simulink model "model_8264"  (R2022b)
settings: Solver=FixedStepAuto  StartTime=0.0  StopTime=2.4  FixedStep=2e-5  RelTol=1e-3
undefined symbols (not defined in the file): Acid, Lead, sigbuilder_block
libraries: spsMeanLib x24, spsVoltageMeasurementLib x18, spsGroundLib x15, spsCurrentMeasurementLib x15, spsIdealSwitchLib x12, spsSeriesRLCLoadLib x12, spsSeriesRLCBranchLib x5, spsThreePhaseVIMeasurementLib x4, simulink x4, spsPower3phInstantaneousLib x3, spsThreePhaseBreakerLib x2, slpidlib x2
(part 1 of 2)
settings Model: Creator=LiChao  LastModifiedBy=ldt20
settings ModelReferenceCC: EnableRefExpFcnMdlSchedulingChecks=on

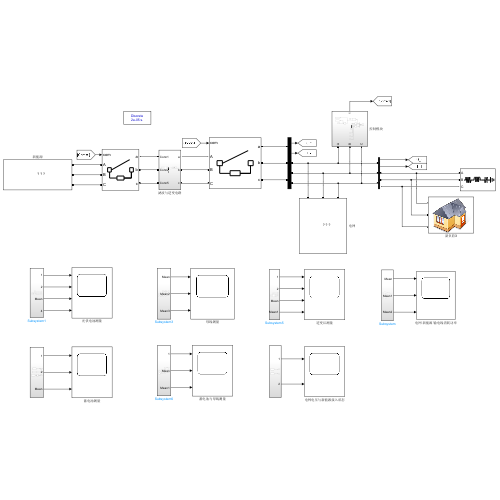
[thumbnail: Simulink's stored preview of the top-level diagram]
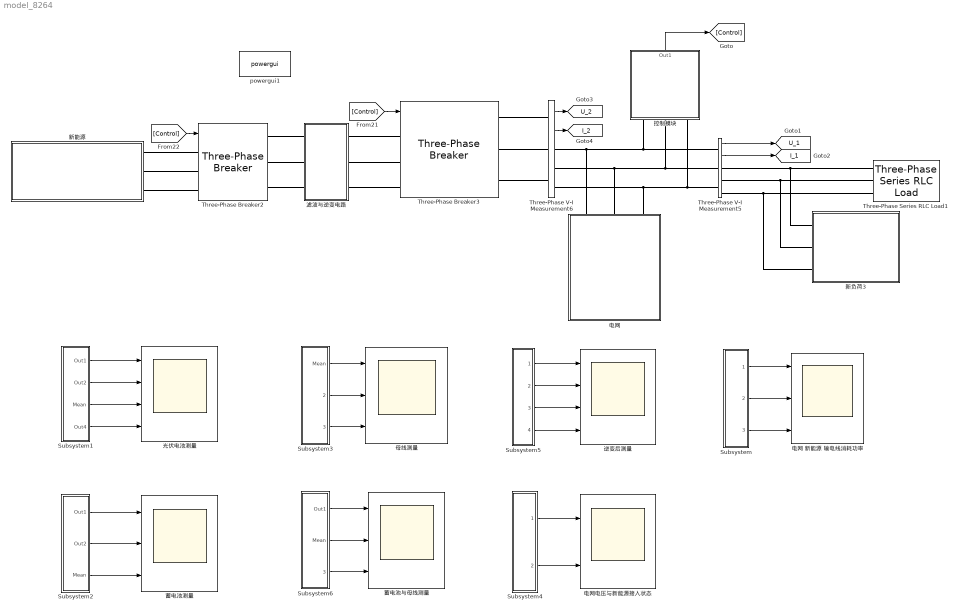
== system model_8264 ==
  Subsystem : Subsystem
  Subsystem1 : Subsystem
  Subsystem2 : Subsystem
  Subsystem3 : Subsystem
  Subsystem4 : Subsystem
  Subsystem5 : Subsystem
  Subsystem6 : Subsystem
  Three-Phase Series RLC Load1 : spsThreePhaseSeriesRLCLoadLib/Three-Phase Series RLC Load  LConnTagsString=A|B|C  Configuration=Y (grounded)  NominalVoltage=1000  Vabc=[1e3 1e3 1e3]  Vabcp=[1e3 1e3 1e3]  NominalFrequency=50  UnbalancedPower=off  ActivePower=1  InductivePower=100  CapacitivePower=100  Pabc=[10e3 9e3 11e3]  QLabc=[100 90 110]  QCabc=[100 90 110]  Pabcp=[10e3 9e3 11e3]  QLabcp=[100 90 110]  QCabcp=[100 90 110]  Measurements=None  LoadType=constant Z
  Three-Phase V-I Measurement5 : spsThreePhaseVIMeasurementLib/Three-Phase V-I Measurement  VoltageMeasurement=phase-to-ground  SetLabelV=off  LabelV=Vgrid0  Vpu=off  VpuLL=off  CurrentMeasurement=yes  SetLabelI=off  LabelI=Igrid  Ipu=off  Pbase=100e6  Vbase=500e3  OutputType=Complex  PhasorSimulation=off  PSBequivalent=0
  Three-Phase V-I Measurement6 : spsThreePhaseVIMeasurementLib/Three-Phase V-I Measurement  VoltageMeasurement=phase-to-ground  SetLabelV=off  LabelV=Vgrid0  Vpu=off  VpuLL=off  CurrentMeasurement=yes  SetLabelI=off  LabelI=Igrid  Ipu=off  Pbase=100e6  Vbase=500e3  OutputType=Complex  PhasorSimulation=off  PSBequivalent=0
  Three-Phase Breaker2 : spsThreePhaseBreakerLib/Three-Phase Breaker  InitialState=open  SwitchA=on  SwitchB=on  SwitchC=on  SwitchTimes="[1/60  5/60]"  External=on  BreakerResistance=0.01  SnubberResistance=1e6  SnubberCapacitance=inf  Measurements=None
  Three-Phase Breaker3 : spsThreePhaseBreakerLib/Three-Phase Breaker  InitialState=open  SwitchA=on  SwitchB=on  SwitchC=on  SwitchTimes="[1/60  5/60]"  External=on  BreakerResistance=0.01  SnubberResistance=1e6  SnubberCapacitance=inf  Measurements=None
  powergui1 : spspowerguiLib/powergui  Priority=1  SimulationMode=Discrete  SampleTime=2e-5  frequency=60  Iterations=50  frequencyindice=0  Pbase=100e6  ErrMax=1e-4  UnitsV=kV  UnitsW=MW  buscounter=0  FunctionMessages=off  echomessages=off  EnableUseOfTLC=off  CurrentSourceSwitches=off  DisableSnubberDevices=off  DisableRonSwitches=off  DisableVfSwitches=off  DisplayEquations=off  AutomaticDiscreteSolvers=off  SolverType=Tustin/Backward Euler (TBE)  Interpol=off  ExternalGateDelay=off  methode=off  Ts=100  x0status=blocks  SPID=on  SwTol=0  HookPort=off  NonlinearTolerance=1e-4  nMaxIteration=100  ContinueOnMaxIteration=off  RestoreLinks=warning  ResistiveCurrentMeasurement=off  Frange=[0:2:500]  Ylog=off  Xlog=on  ShowGrid=off  save=off  variable=ZData  structure=0  ZoomFFT=off  StartTime=0.0  cycles=1  DisplayStyle=1  fundamental=60  FreqAxis=off  MaxFrequency=1000  frequencyindicesteady=1  RmsSteady=1  display=off
  光伏电池测量 : Scope  NumInputPorts=4
  控制模块 : Subsystem
  新能源 : Subsystem
      mask Display: image('xinengyuan.jpg'); % 使用工具条上的 "编辑图像" 进行更改。
  新负荷3 : Subsystem
      mask Display: image('house.jpg'); % 使用工具条上的 "编辑图像" 进行更改。
  母线测量 : Scope  NumInputPorts=3
  滤波与逆变电路 : Subsystem
  电网 : Subsystem
      mask Display: image('dianwang.jpg'); % 使用工具条上的 "编辑图像" 进行更改。
  电网 新能源 输电线消耗功率 : Scope  NumInputPorts=3
  电网电压与新能源接入状态 : Scope  NumInputPorts=2
  蓄电池与母线测量 : Scope  NumInputPorts=3
  蓄电池测量 : Scope  NumInputPorts=3
  逆变后测量 : Scope  NumInputPorts=4
  tag scope: I_1=global, I_2=global, U_1=global, U_2=global
  wires:
  控制模块/1(Out1) -> [Control]
  [Control] -> Three-Phase Breaker3/1
  [Control] -> Three-Phase Breaker2/1
  Three-Phase V-I Measurement5/1 -> [U_1]
  Three-Phase V-I Measurement5/2 -> [I_1]
  Three-Phase V-I Measurement6/1 -> [U_2]
  Three-Phase V-I Measurement6/2 -> [I_2]
  Subsystem/1(Mean) -> 电网 新能源 输电线消耗功率/1
  Subsystem/2(Mean1) -> 电网 新能源 输电线消耗功率/2
  Subsystem/3(Mean2) -> 电网 新能源 输电线消耗功率/3
  Subsystem1/1(Out1) -> 光伏电池测量/1
  Subsystem1/2(Out2) -> 光伏电池测量/2
  Subsystem1/3(Mean) -> 光伏电池测量/3
  Subsystem1/4(Out4) -> 光伏电池测量/4
  Subsystem2/1(Out1) -> 蓄电池测量/1
  Subsystem2/2(Out2) -> 蓄电池测量/2
  Subsystem2/3(Mean) -> 蓄电池测量/3
  Subsystem3/1(Mean) -> 母线测量/1
  Subsystem3/2(Mean2) -> 母线测量/2
  Subsystem3/3(Mean3) -> 母线测量/3
  Subsystem4/1(Out1) -> 电网电压与新能源接入状态/1
  Subsystem4/2(Out2) -> 电网电压与新能源接入状态/2
  Subsystem5/1(Out1) -> 逆变后测量/1
  Subsystem5/2(Out2) -> 逆变后测量/2
  Subsystem5/3(Mean) -> 逆变后测量/3
  Subsystem5/4(Mean1) -> 逆变后测量/4
  Subsystem6/1(Out1) -> 蓄电池与母线测量/1
  Subsystem6/2(Mean) -> 蓄电池与母线测量/2
  Subsystem6/3(Mean1) -> 蓄电池与母线测量/3
  connections:
  Three-Phase Breaker3/LConn1 -- 滤波与逆变电路/RConn1
  Three-Phase Breaker2/RConn2 -- 滤波与逆变电路/LConn2
  Three-Phase Breaker3/LConn2 -- 滤波与逆变电路/RConn2
  新能源/LConn1 -- Three-Phase Breaker2/LConn1
  Three-Phase Breaker3/LConn3 -- 滤波与逆变电路/RConn3
  新能源/LConn2 -- Three-Phase Breaker2/LConn2
  Three-Phase Breaker2/RConn3 -- 滤波与逆变电路/LConn3
  Three-Phase V-I Measurement6/LConn2 -- Three-Phase Breaker3/RConn2
  新能源/LConn3 -- Three-Phase Breaker2/LConn3
  Three-Phase V-I Measurement6/LConn3 -- Three-Phase Breaker3/RConn3
  Three-Phase Breaker2/RConn1 -- 滤波与逆变电路/LConn1
  Three-Phase V-I Measurement6/LConn1 -- Three-Phase Breaker3/RConn1
  Three-Phase V-I Measurement6/RConn1 -- 电网/RConn1 -- 控制模块/LConn1 -- Three-Phase V-I Measurement5/LConn1
  Three-Phase V-I Measurement6/RConn2 -- 电网/RConn2 -- 控制模块/LConn2 -- Three-Phase V-I Measurement5/LConn2
  Three-Phase V-I Measurement6/RConn3 -- 电网/RConn3 -- Three-Phase V-I Measurement5/LConn3 -- 控制模块/LConn3
  Three-Phase V-I Measurement5/RConn1 -- 新负荷3/LConn1 -- Three-Phase Series RLC Load1/LConn1
  Three-Phase V-I Measurement5/RConn2 -- 新负荷3/LConn2 -- Three-Phase Series RLC Load1/LConn2
  Three-Phase V-I Measurement5/RConn3 -- 新负荷3/LConn3 -- Three-Phase Series RLC Load1/LConn3

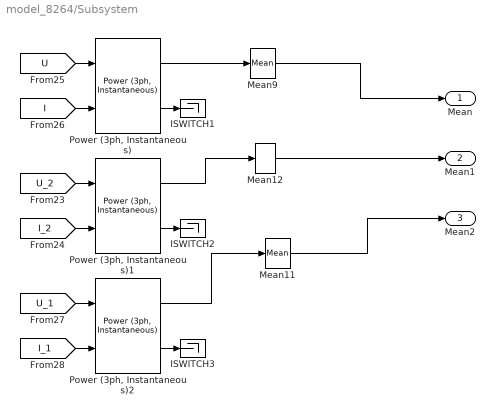
== system model_8264/Subsystem ==
  ISWITCH1 : Terminator
  ISWITCH2 : Terminator
  ISWITCH3 : Terminator
  Mean11 : spsMeanLib/Mean  Freq=50  Vinit=0  Ts=0
  Mean12 : spsMeanLib/Mean  Freq=50  Vinit=0  Ts=0
  Mean9 : spsMeanLib/Mean  Freq=50  Vinit=0  Ts=0
  "Power (3ph, Instantaneous)" : spsPower3phInstantaneousLib/Power (3ph, Instantaneous)
  "Power (3ph, Instantaneous)1" : spsPower3phInstantaneousLib/Power (3ph, Instantaneous)
  "Power (3ph, Instantaneous)2" : spsPower3phInstantaneousLib/Power (3ph, Instantaneous)
  Mean : Outport
  Mean1 : Outport  Port=2
  Mean2 : Outport  Port=3
  wires:
  Mean11/1 -> Mean2/1
  [I_1] -> "Power (3ph, Instantaneous)2"/2
  "Power (3ph, Instantaneous)2"/1 -> Mean11/1
  [U_2] -> "Power (3ph, Instantaneous)1"/1
  "Power (3ph, Instantaneous)1"/1 -> Mean12/1
  [U_1] -> "Power (3ph, Instantaneous)2"/1
  Mean12/1 -> Mean1/1
  [U] -> "Power (3ph, Instantaneous)"/1
  "Power (3ph, Instantaneous)"/1 -> Mean9/1
  [I] -> "Power (3ph, Instantaneous)"/2
  [I_2] -> "Power (3ph, Instantaneous)1"/2
  "Power (3ph, Instantaneous)2"/2 -> ISWITCH3/1
  "Power (3ph, Instantaneous)1"/2 -> ISWITCH2/1
  Mean9/1 -> Mean/1
  "Power (3ph, Instantaneous)"/2 -> ISWITCH1/1

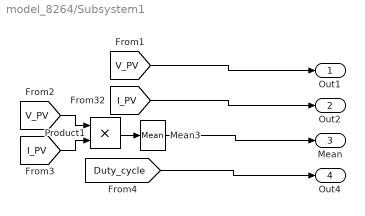
== system model_8264/Subsystem1 ==
  Mean3 : spsMeanLib/Mean  Freq=50  Vinit=0  Ts=0
  Product1 : Product
  Out1 : Outport
  Out2 : Outport  Port=2
  Mean : Outport  Port=3
  Out4 : Outport  Port=4
  wires:
  Product1/1 -> Mean3/1
  [V_PV] -> Product1/1
  Mean3/1 -> Mean/1
  [I_PV] -> Out2/1
  [Duty_cycle] -> Out4/1
  [I_PV] -> Product1/2
  [V_PV] -> Out1/1

== system model_8264/Subsystem2 ==
  Mean7 : spsMeanLib/Mean  Freq=50  Vinit=0  Ts=0
  Out1 : Outport
  Out2 : Outport  Port=2
  Mean : Outport  Port=3
  wires:
  [I_battery] -> Mean7/1
  [SOC] -> Out1/1
  Mean7/1 -> Mean/1
  [U_battery] -> Out2/1

== system model_8264/Subsystem3 ==
  Mean1 : spsMeanLib/Mean  Freq=50  Vinit=0  Ts=0
  Mean6 : spsMeanLib/Mean  Freq=50  Vinit=0  Ts=0
  Mean8 : spsMeanLib/Mean  Freq=50  Vinit=0  Ts=0
  Product2 : Product
  Mean : Outport
  Mean2 : Outport  Port=2
  Mean3 : Outport  Port=3
  wires:
  [I_BUS] -> Mean8/1
  [U_BUS] -> Mean6/1
  Mean8/1 -> Mean2/1
  [I_BUS] -> Product2/2
  Mean6/1 -> Mean/1
  Product2/1 -> Mean1/1
  [U_BUS] -> Product2/1
  Mean1/1 -> Mean3/1

== system model_8264/Subsystem4 ==
  Out1 : Outport
  Out2 : Outport  Port=2
  wires:
  [Grid_voltage] -> Out1/1
  [State] -> Out2/1

== system model_8264/Subsystem5 ==
  Mean4 : spsMeanLib/Mean  Freq=50  Vinit=0  Ts=0
  Mean5 : spsMeanLib/Mean  Freq=50  Vinit=0  Ts=0
  "Power (3ph, Phasor)2" : spsPower3phPhasorLib/Power (3ph, Phasor)
  Out1 : Outport
  Out2 : Outport  Port=2
  Mean : Outport  Port=3
  Mean1 : Outport  Port=4
  wires:
  Mean5/1 -> Mean1/1
  [U_ABC] -> "Power (3ph, Phasor)2"/1
  [I_ABC] -> Out2/1
  [I_ABC] -> "Power (3ph, Phasor)2"/2
  "Power (3ph, Phasor)2"/1 -> Mean4/1
  "Power (3ph, Phasor)2"/2 -> Mean5/1
  [U_ABC] -> Out1/1
  Mean4/1 -> Mean/1

== system model_8264/Subsystem6 ==
  Mean10 : spsMeanLib/Mean  Freq=50  Vinit=0  Ts=0
  Mean2 : spsMeanLib/Mean  Freq=50  Vinit=0  Ts=0
  Product3 : Product
  Out1 : Outport
  Mean : Outport  Port=2
  Mean1 : Outport  Port=3
  wires:
  [I_CM] -> Product3/2
  [U_BUS] -> Product3/1
  Product3/1 -> Mean2/1
  [I_CM] -> Mean10/1
  Mean2/1 -> Mean1/1
  Mean10/1 -> Mean/1
  [U_BUS] -> Out1/1

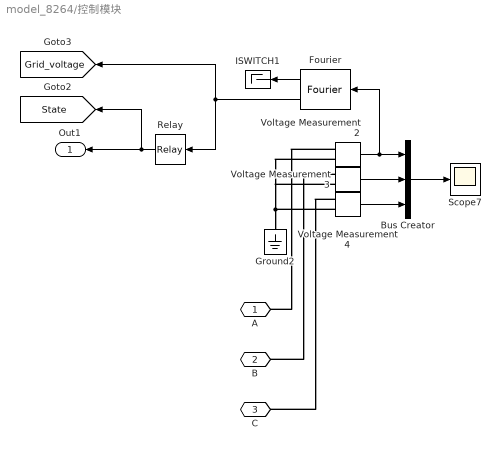
== system model_8264/控制模块 ==
  Bus Creator : BusCreator  Inputs=3
  Fourier : spsFourierLib/Fourier  Freq=50  n=1  InInit=[0, 0]  Ts=0
  Ground2 : spsGroundLib/Ground  LConnTagsString=a
  ISWITCH1 : Terminator
  Relay : Relay  OnSwitchValue=218  OffSwitchValue=215  OnOutputValue=0  OffOutputValue=1
  Scope7 : Scope
  Voltage Measurement2 : spsVoltageMeasurementLib/Voltage Measurement  PhasorSimulation=off  OutputType=Complex  PSBequivalent=0
  Voltage Measurement3 : spsVoltageMeasurementLib/Voltage Measurement  PhasorSimulation=off  OutputType=Complex  PSBequivalent=0
  Voltage Measurement4 : spsVoltageMeasurementLib/Voltage Measurement  PhasorSimulation=off  OutputType=Complex  PSBequivalent=0
  A : PMIOPort  Side=Left
  B : PMIOPort  Port=2  Side=Left
  C : PMIOPort  Port=3  Side=Left
  Out1 : Outport
  tag scope: Grid_voltage=global, State=global
  wires:
  Voltage Measurement2/1 -> Fourier/1, Bus Creator/1
  Fourier/2 -> ISWITCH1/1
  Bus Creator/1 -> Scope7/1
  Relay/1 -> [State], Out1/1
  Fourier/1 -> [Grid_voltage], Relay/1
  Voltage Measurement4/1 -> Bus Creator/3
  Voltage Measurement3/1 -> Bus Creator/2
  connections:
  Voltage Measurement4/LConn2 -- Voltage Measurement2/LConn2 -- Voltage Measurement3/LConn2 -- Ground2/LConn1
  Voltage Measurement4/LConn1 -- C/RConn1
  Voltage Measurement3/LConn1 -- B/RConn1
  Voltage Measurement2/LConn1 -- A/RConn1

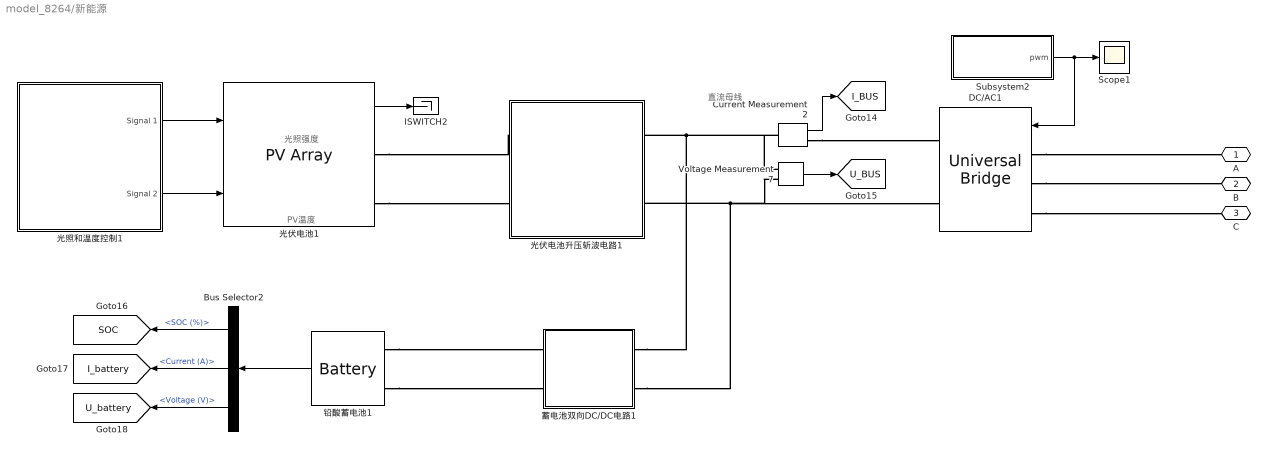
== system model_8264/新能源 ==
  note: 光照强度
  note: PV温度
  note: 直流母线
  Bus Selector2 : BusSelector  OutputSignals=SOC (%),Current (A),Voltage (V)
  Current Measurement2 : spsCurrentMeasurementLib/Current Measurement  PhasorSimulation=off  OutputType=Complex  PSBequivalent=0
  DC/AC1 : spsUniversalBridgeLib/Universal Bridge  Arms=3  SnubberResistance=1e5  SnubberCapacitance=inf  Device=IGBT / Diodes  Ron=1e-3  Lon=0  ForwardVoltages="[  0  0  ]"  ForwardVoltage=0  GTOparameters=[ 10e-6 , 20e-6 ]  IGBTparameters=[ 1e-6 , 2e-6 ]  Measurements=None  Measurements_2=None  converterType=Rectifier
  ISWITCH2 : Terminator
  Scope1 : Scope
  Subsystem2 : Subsystem  mask{m=0.8, fc=100000000, f=50}
      mask prompts: m "m(0<m<=1)"
  Voltage Measurement7 : spsVoltageMeasurementLib/Voltage Measurement  PhasorSimulation=off  OutputType=Complex  PSBequivalent=0
  光伏电池1 : spsPVArrayLib/PV Array  Npar=2  Nser=10  PlotType=array @ 1000 W/m2 & specified temperatures  S_vec="[ 1000  500  100 ]"  Temp_C_vec="[ 45 25  ]"  ModuleName=User-defined  PlotWhenSelected=off  Pm=120.7  Ncell=72  Voc=21  Isc=8  Vm=17  Im=7.1  beta_Voc_pc=-0.358  alpha_Isc_pc=0.052  beta_Voc=-0.07518  alpha_Isc=0.00416  IL=8.0496  I0=2.4168e-10  nI=0.47021  Rsh=31.6334  Rs=0.196  RobustModel=off  RobustCellTemperature=313.3991  BAL=off  Tc=1e-6  Tfilter=5e-5
  光伏电池升压斩波电路1 : Subsystem
  光照和温度控制1 : Subsystem  Tag=STV Subsys  LoadFcn=sigbuilder_block('load');  StartFcn=sigbuilder_block('start');  StopFcn=sigbuilder_block('stop');  ClipboardFcn=sigbuilder_block('clipboard');  mask(Sigbuilder block){tuvar=[0:10]}
      mask help: Simulink:masks:SigbuilderBlock_MD
      mask init:
      | if ~strcmp(get_param(bdroot(gcbh),'SimulationStatus'),'stopped') tuvar = sigbuilder_block('maskInit'); end
      settings: CopyFcn=sigbuilder_block('copy');  DeleteFcn=sigbuilder_block('delete');  ModelCloseFcn=sigbuilder_block('modelClose');  PreSaveFcn=sigbuilder_block('preSave');  PauseFcn=sigbuilder_block('pause');  ContinueFcn=sigbuilder_block('continue');  NameChangeFcn=sigbuilder_block('namechange');  OpenFcn=sigbuilder_block('open',[122 118.5 1141 444 ]);  CloseFcn=sigbuilder_block('close');
      mask Display: plot(0, 0, 100, 100,[2, 2, 32, 32, 2], [68, 8, 8, 68, 68],[32, 2], [38, 38], [32, 19, 2],[53, 60, 44], [32, 17, 17, 2],[16, 16, 31, 31]);txt = getActiveGroup(gcbh);text(2, 100, txt,'verticalAlignment', 'top');
  蓄电池双向DC/DC电路1 : Subsystem
  铅酸蓄电池1 : spsBatteryLib/Battery  BatType=Lead-Acid  ShowTempParam=off  ThermalPreset=no  ShowAgeParam=off  NomV=250  NomQ=50  SOC=80  Batt_Tr=30  PresetModel=on  MaxQ=52.0833  MinV=187.5  FullV=272.2039  Dis_rate=10  R=0.05  Normal_OP=15.5139  expZone="[254.523     0.1666667]"  current=[6.5 13 32.5]  Units=Time  Tci=20  NomT=20  T2=-30  MaxQ2=4.8  FullV2=7.1  Normal_OP2=5.655  expZone2="[6.58           1]"  Rca=0.6  ti=2000  Dp=0  Neq0=0  Tsim=1e6  Ta1=25  Qeol=5.4*0.9  Reol=0.013333*1.2  Char_age=[2.3478, 3]  Dis_age=[2.3478, 10]  N1=1500  N2=10500  N3=1000  N4=1400  Ta2=45  N5=950
  A : PMIOPort  Side=Left
  B : PMIOPort  Port=2  Side=Left
  C : PMIOPort  Port=3  Side=Left
  tag scope: I_BUS=global, I_battery=global, SOC=global, U_BUS=global, U_battery=global
  wires:
  Subsystem2/1(pwm) -> DC/AC1/1, Scope1/1
  铅酸蓄电池1/1 -> Bus Selector2/1
  Bus Selector2/3 -> [U_battery]  "<Voltage (V)>"
  Voltage Measurement7/1 -> [U_BUS]
  Current Measurement2/1 -> [I_BUS]
  光伏电池1/1 -> ISWITCH2/1
  Bus Selector2/1 -> [SOC]  "<SOC (%)>"
  光照和温度控制1/1(Signal 1) -> 光伏电池1/1
  光照和温度控制1/2(Signal 2) -> 光伏电池1/2
  Bus Selector2/2 -> [I_battery]  "<Current (A)>"
  connections:
  蓄电池双向DC/DC电路1/RConn2 -- 光伏电池升压斩波电路1/RConn2 -- DC/AC1/RConn2 -- Voltage Measurement7/LConn2
  光伏电池1/RConn2 -- 光伏电池升压斩波电路1/LConn2
  蓄电池双向DC/DC电路1/RConn1 -- 光伏电池升压斩波电路1/RConn1 -- Voltage Measurement7/LConn1 -- Current Measurement2/LConn1
  DC/AC1/LConn1 -- A/RConn1
  铅酸蓄电池1/LConn2 -- 蓄电池双向DC/DC电路1/LConn2
  DC/AC1/LConn3 -- C/RConn1
  光伏电池1/RConn1 -- 光伏电池升压斩波电路1/LConn1
  DC/AC1/LConn2 -- B/RConn1
  Current Measurement2/RConn1 -- DC/AC1/RConn1
  铅酸蓄电池1/LConn1 -- 蓄电池双向DC/DC电路1/LConn1

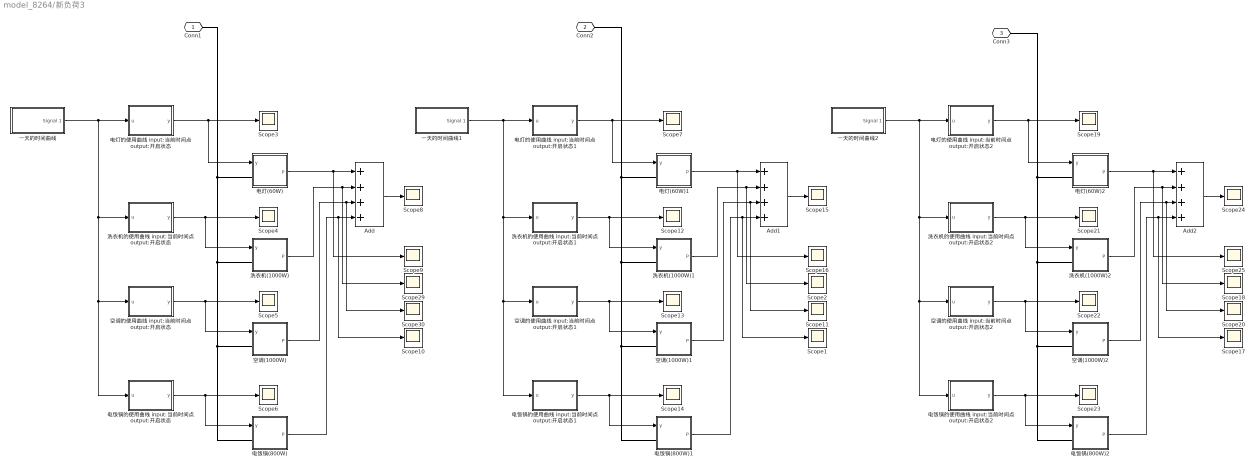
== system model_8264/新负荷3 ==
  Add : Sum  Inputs=++++
  Add1 : Sum  Inputs=++++
  Add2 : Sum  Inputs=++++
  Scope{1..25,29..30} (27 alike) : Scope
  一天的时间曲线 : Subsystem  Tag=STV Subsys  LoadFcn=sigbuilder_block('load');  StartFcn=sigbuilder_block('start');  StopFcn=sigbuilder_block('stop');  ClipboardFcn=sigbuilder_block('clipboard');  mask(Sigbuilder block){tuvar=[0:10]}
      mask help: Simulink:masks:SigbuilderBlock_MD
      mask init:
      | if ~strcmp(get_param(bdroot(gcbh),'SimulationStatus'),'stopped') tuvar = sigbuilder_block('maskInit'); end
      settings: CopyFcn=sigbuilder_block('copy');  DeleteFcn=sigbuilder_block('delete');  ModelCloseFcn=sigbuilder_block('modelClose');  PreSaveFcn=sigbuilder_block('preSave');  PauseFcn=sigbuilder_block('pause');  ContinueFcn=sigbuilder_block('continue');  NameChangeFcn=sigbuilder_block('namechange');  OpenFcn=sigbuilder_block('open',[348.6 91.2 550.8 400.2 ]);  CloseFcn=sigbuilder_block('close');
      mask Display: plot(0, 0, 100, 100,[2, 2, 32, 32, 2], [68, 8, 8, 68, 68],[32, 2], [38, 38], [32, 19, 2],[53, 60, 44], [32, 17, 17, 2],[16, 16, 31, 31]);txt = getActiveGroup(gcbh);text(2, 100, txt,'verticalAlignment', 'top');
  一天的时间曲线1 : Subsystem  Tag=STV Subsys  LoadFcn=sigbuilder_block('load');  StartFcn=sigbuilder_block('start');  StopFcn=sigbuilder_block('stop');  ClipboardFcn=sigbuilder_block('clipboard');  mask(Sigbuilder block){tuvar=[0:10]}
      mask help: Simulink:masks:SigbuilderBlock_MD
      mask init:
      | if ~strcmp(get_param(bdroot(gcbh),'SimulationStatus'),'stopped') tuvar = sigbuilder_block('maskInit'); end
      settings: CopyFcn=sigbuilder_block('copy');  DeleteFcn=sigbuilder_block('delete');  ModelCloseFcn=sigbuilder_block('modelClose');  PreSaveFcn=sigbuilder_block('preSave');  PauseFcn=sigbuilder_block('pause');  ContinueFcn=sigbuilder_block('continue');  NameChangeFcn=sigbuilder_block('namechange');  OpenFcn=sigbuilder_block('open',[348.6 91.2 550.8 400.2 ]);  CloseFcn=sigbuilder_block('close');
      mask Display: plot(0, 0, 100, 100,[2, 2, 32, 32, 2], [68, 8, 8, 68, 68],[32, 2], [38, 38], [32, 19, 2],[53, 60, 44], [32, 17, 17, 2],[16, 16, 31, 31]);txt = getActiveGroup(gcbh);text(2, 100, txt,'verticalAlignment', 'top');
  一天的时间曲线2 : Subsystem  Tag=STV Subsys  LoadFcn=sigbuilder_block('load');  StartFcn=sigbuilder_block('start');  StopFcn=sigbuilder_block('stop');  ClipboardFcn=sigbuilder_block('clipboard');  mask(Sigbuilder block){tuvar=[0:10]}
      mask help: Simulink:masks:SigbuilderBlock_MD
      mask init:
      | if ~strcmp(get_param(bdroot(gcbh),'SimulationStatus'),'stopped') tuvar = sigbuilder_block('maskInit'); end
      settings: CopyFcn=sigbuilder_block('copy');  DeleteFcn=sigbuilder_block('delete');  ModelCloseFcn=sigbuilder_block('modelClose');  PreSaveFcn=sigbuilder_block('preSave');  PauseFcn=sigbuilder_block('pause');  ContinueFcn=sigbuilder_block('continue');  NameChangeFcn=sigbuilder_block('namechange');  OpenFcn=sigbuilder_block('open',[348.6 91.2 550.8 400.2 ]);  CloseFcn=sigbuilder_block('close');
      mask Display: plot(0, 0, 100, 100,[2, 2, 32, 32, 2], [68, 8, 8, 68, 68],[32, 2], [38, 38], [32, 19, 2],[53, 60, 44], [32, 17, 17, 2],[16, 16, 31, 31]);txt = getActiveGroup(gcbh);text(2, 100, txt,'verticalAlignment', 'top');
  洗衣机(1000W) : Subsystem
  洗衣机(1000W)1 : Subsystem
  洗衣机(1000W)2 : Subsystem
  洗衣机的使用曲线 input:当前时间点 output:开启状态 : MATLAB Function  TreatAsAtomicUnit=on
  洗衣机的使用曲线 input:当前时间点 output:开启状态1 : MATLAB Function  TreatAsAtomicUnit=on
  洗衣机的使用曲线 input:当前时间点 output:开启状态2 : MATLAB Function  TreatAsAtomicUnit=on
  电灯(60W) : Subsystem
  电灯(60W)1 : Subsystem
  电灯(60W)2 : Subsystem
  电灯的使用曲线 input:当前时间点 output:开启状态 : MATLAB Function  TreatAsAtomicUnit=on
  电灯的使用曲线 input:当前时间点 output:开启状态1 : MATLAB Function  TreatAsAtomicUnit=on
  电灯的使用曲线 input:当前时间点 output:开启状态2 : MATLAB Function  TreatAsAtomicUnit=on
  电饭锅(800W) : Subsystem
  电饭锅(800W)1 : Subsystem
  电饭锅(800W)2 : Subsystem
  电饭锅的使用曲线 input:当前时间点 output:开启状态 : MATLAB Function  TreatAsAtomicUnit=on
  电饭锅的使用曲线 input:当前时间点 output:开启状态1 : MATLAB Function  TreatAsAtomicUnit=on
  电饭锅的使用曲线 input:当前时间点 output:开启状态2 : MATLAB Function  TreatAsAtomicUnit=on
  空调(1000W) : Subsystem
  空调(1000W)1 : Subsystem
  空调(1000W)2 : Subsystem
  空调的使用曲线 input:当前时间点 output:开启状态 : MATLAB Function  TreatAsAtomicUnit=on
  空调的使用曲线 input:当前时间点 output:开启状态1 : MATLAB Function  TreatAsAtomicUnit=on
  空调的使用曲线 input:当前时间点 output:开启状态2 : MATLAB Function  TreatAsAtomicUnit=on
  Conn2 : PMIOPort  Port=2  Side=Left
  Conn3 : PMIOPort  Port=3  Side=Left
  Conn1 : PMIOPort  Side=Left
  wires:
  空调的使用曲线 input:当前时间点 output:开启状态/1(y) -> 空调(1000W)/1(y), Scope5/1
  洗衣机的使用曲线 input:当前时间点 output:开启状态/1(y) -> 洗衣机(1000W)/1(y), Scope4/1
  电灯的使用曲线 input:当前时间点 output:开启状态/1(y) -> 电灯(60W)/1(y), Scope3/1
  电饭锅(800W)/1(P) -> Scope10/1, Add/4
  空调(1000W)/1(P) -> Scope30/1, Add/3
  Add/1 -> Scope8/1
  电饭锅的使用曲线 input:当前时间点 output:开启状态/1(y) -> 电饭锅(800W)/1(y), Scope6/1
  一天的时间曲线/1(Signal 1) -> 电饭锅的使用曲线 input:当前时间点 output:开启状态/1(u), 空调的使用曲线 input:当前时间点 output:开启状态/1(u), 洗衣机的使用曲线 input:当前时间点 output:开启状态/1(u), 电灯的使用曲线 input:当前时间点 output:开启状态/1(u)
  电灯(60W)/1(P) -> Scope9/1, Add/1
  洗衣机(1000W)/1(P) -> Scope29/1, Add/2
  洗衣机(1000W)1/1(P) -> Scope2/1, Add1/2
  电饭锅(800W)1/1(P) -> Scope1/1, Add1/4
  电饭锅的使用曲线 input:当前时间点 output:开启状态1/1(y) -> 电饭锅(800W)1/1(y), Scope14/1
  电灯的使用曲线 input:当前时间点 output:开启状态1/1(y) -> 电灯(60W)1/1(y), Scope7/1
  一天的时间曲线1/1(Signal 1) -> 电饭锅的使用曲线 input:当前时间点 output:开启状态1/1(u), 空调的使用曲线 input:当前时间点 output:开启状态1/1(u), 洗衣机的使用曲线 input:当前时间点 output:开启状态1/1(u), 电灯的使用曲线 input:当前时间点 output:开启状态1/1(u)
  电灯(60W)1/1(P) -> Scope16/1, Add1/1
  Add1/1 -> Scope15/1
  空调(1000W)1/1(P) -> Scope11/1, Add1/3
  洗衣机的使用曲线 input:当前时间点 output:开启状态1/1(y) -> 洗衣机(1000W)1/1(y), Scope12/1
  空调的使用曲线 input:当前时间点 output:开启状态1/1(y) -> 空调(1000W)1/1(y), Scope13/1
  洗衣机(1000W)2/1(P) -> Scope18/1, Add2/2
  电饭锅(800W)2/1(P) -> Scope17/1, Add2/4
  电饭锅的使用曲线 input:当前时间点 output:开启状态2/1(y) -> 电饭锅(800W)2/1(y), Scope23/1
  电灯的使用曲线 input:当前时间点 output:开启状态2/1(y) -> 电灯(60W)2/1(y), Scope19/1
  一天的时间曲线2/1(Signal 1) -> 电饭锅的使用曲线 input:当前时间点 output:开启状态2/1(u), 空调的使用曲线 input:当前时间点 output:开启状态2/1(u), 洗衣机的使用曲线 input:当前时间点 output:开启状态2/1(u), 电灯的使用曲线 input:当前时间点 output:开启状态2/1(u)
  电灯(60W)2/1(P) -> Scope25/1, Add2/1
  Add2/1 -> Scope24/1
  空调(1000W)2/1(P) -> Scope20/1, Add2/3
  洗衣机的使用曲线 input:当前时间点 output:开启状态2/1(y) -> 洗衣机(1000W)2/1(y), Scope21/1
  空调的使用曲线 input:当前时间点 output:开启状态2/1(y) -> 空调(1000W)2/1(y), Scope22/1
  connections:
  电饭锅(800W)/LConn1 -- 空调(1000W)/LConn1 -- 洗衣机(1000W)/LConn1 -- 电灯(60W)/LConn1 -- Conn1/RConn1
  电饭锅(800W)1/LConn1 -- 空调(1000W)1/LConn1 -- 洗衣机(1000W)1/LConn1 -- 电灯(60W)1/LConn1 -- Conn2/RConn1
  电饭锅(800W)2/LConn1 -- 空调(1000W)2/LConn1 -- 洗衣机(1000W)2/LConn1 -- 电灯(60W)2/LConn1 -- Conn3/RConn1

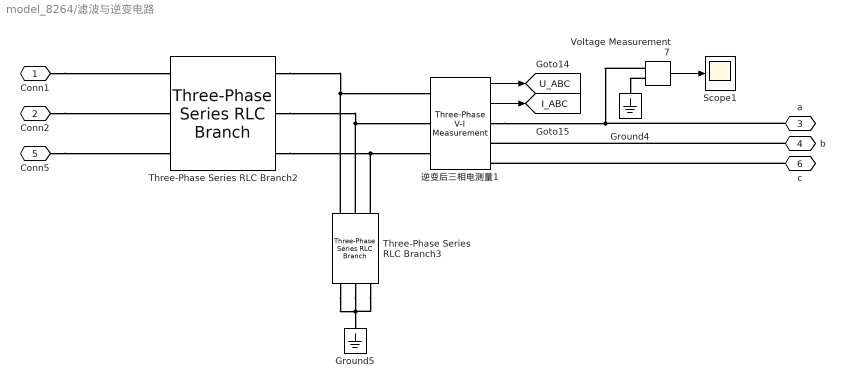
== system model_8264/滤波与逆变电路 ==
  Ground4 : spsGroundLib/Ground  LConnTagsString=a
  Ground5 : spsGroundLib/Ground  LConnTagsString=a
  Scope1 : Scope
  Three-Phase Series RLC Branch2 : spsThreePhaseSeriesRLCBranchLib/Three-Phase Series RLC Branch  LConnTagsString=A|B|C  RConnTagsString=A|B|C  BranchType=L  Resistance=0.01  Inductance=0.001  Capacitance=1e-6  Measurements=None
  Three-Phase Series RLC Branch3 : spsThreePhaseSeriesRLCBranchLib/Three-Phase Series RLC Branch  LConnTagsString=A|B|C  RConnTagsString=A|B|C  BranchType=C  Resistance=1  Inductance=1e-3  Capacitance=1e-5  Measurements=None
  Voltage Measurement7 : spsVoltageMeasurementLib/Voltage Measurement  PhasorSimulation=off  OutputType=Complex  PSBequivalent=0
  逆变后三相电测量1 : spsThreePhaseVIMeasurementLib/Three-Phase V-I Measurement  VoltageMeasurement=phase-to-ground  SetLabelV=off  LabelV=Vabc  Vpu=off  VpuLL=off  CurrentMeasurement=yes  SetLabelI=off  LabelI=Iabc  Ipu=off  Pbase=100e6  Vbase=500e3  OutputType=Complex  PhasorSimulation=off  PSBequivalent=0
  Conn1 : PMIOPort  Side=Left
  Conn2 : PMIOPort  Port=2  Side=Left
  a : PMIOPort  Port=3  Side=Right
  b : PMIOPort  Port=4  Side=Right
  Conn5 : PMIOPort  Port=5  Side=Left
  c : PMIOPort  Port=6  Side=Right
  tag scope: I_ABC=global, U_ABC=global
  wires:
  逆变后三相电测量1/2 -> [I_ABC]
  Voltage Measurement7/1 -> Scope1/1
  逆变后三相电测量1/1 -> [U_ABC]
  connections:
  Three-Phase Series RLC Branch3/LConn2 -- 逆变后三相电测量1/LConn2 -- Three-Phase Series RLC Branch2/RConn2
  c/RConn1 -- 逆变后三相电测量1/RConn3
  Three-Phase Series RLC Branch3/LConn1 -- 逆变后三相电测量1/LConn1 -- Three-Phase Series RLC Branch2/RConn1
  逆变后三相电测量1/RConn1 -- Voltage Measurement7/LConn1 -- a/RConn1
  Voltage Measurement7/LConn2 -- Ground4/LConn1
  Three-Phase Series RLC Branch3/RConn3 -- Ground5/LConn1 -- Three-Phase Series RLC Branch3/RConn2 -- Three-Phase Series RLC Branch3/RConn1
  Three-Phase Series RLC Branch3/LConn3 -- 逆变后三相电测量1/LConn3 -- Three-Phase Series RLC Branch2/RConn3
  Conn1/RConn1 -- Three-Phase Series RLC Branch2/LConn1
  Conn2/RConn1 -- Three-Phase Series RLC Branch2/LConn2
  Conn5/RConn1 -- Three-Phase Series RLC Branch2/LConn3
  b/RConn1 -- 逆变后三相电测量1/RConn2

== system model_8264/电网 ==
  Three-Phase V-I Measurement4 : spsThreePhaseVIMeasurementLib/Three-Phase V-I Measurement  VoltageMeasurement=phase-to-ground  SetLabelV=off  LabelV=Vgrid0  Vpu=off  VpuLL=off  CurrentMeasurement=yes  SetLabelI=off  LabelI=Igrid  Ipu=off  Pbase=100e6  Vbase=500e3  OutputType=Complex  PhasorSimulation=off  PSBequivalent=0
  Three-Phase Source2 : spsThreePhaseSourceLib/Three-Phase Source  InternalConnection=Yg  VoltagePhases=off  Voltage=269.5  PhaseAngle=0  Voltage_phases=[25e3 25e3 25e3]/sqrt(3)  PhaseAngles_phases=[0 -120 +120]  Frequency=50  NonIdealSource=on  SpecifyImpedance=off  Resistance=0.1  Inductance=0  ShortCircuitLevel=100e6  BaseVoltage=25e3  XRratio=7  BusType=swing  Pref=10e3  Qref=0  Prefabc=[10e3, 10e3, 10e3]  Qrefabc=[0, 0, 0]  Qmin=-inf  Qmax=inf
  b : PMIOPort  Port=2  Side=Right
  c : PMIOPort  Port=3  Side=Right
  a : PMIOPort  Side=Right
  tag scope: I=global, U=global
  wires:
  Three-Phase V-I Measurement4/2 -> [I]
  Three-Phase V-I Measurement4/1 -> [U]
  connections:
  Three-Phase V-I Measurement4/RConn1 -- a/RConn1
  Three-Phase V-I Measurement4/RConn2 -- b/RConn1
  Three-Phase Source2/RConn1 -- Three-Phase V-I Measurement4/LConn1
  Three-Phase Source2/RConn3 -- Three-Phase V-I Measurement4/LConn3
  Three-Phase Source2/RConn2 -- Three-Phase V-I Measurement4/LConn2
  Three-Phase V-I Measurement4/RConn3 -- c/RConn1

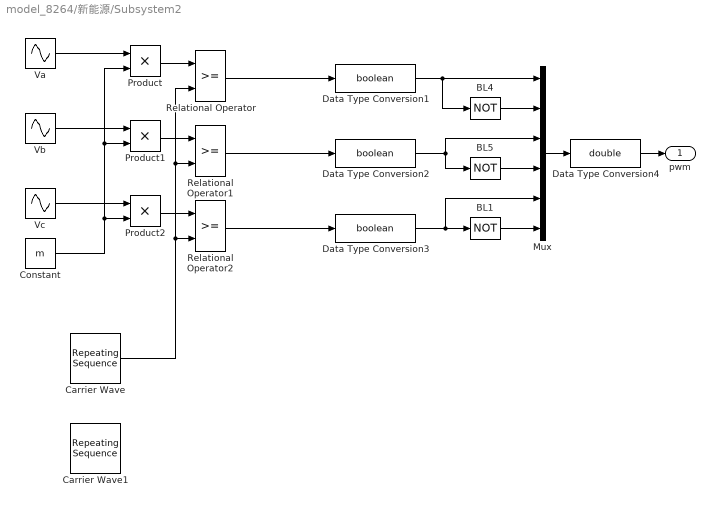
== system model_8264/新能源/Subsystem2 ==
  BL1 : Logic  Operator=NOT  Inputs=1
  BL4 : Logic  Operator=NOT  Inputs=1
  BL5 : Logic  Operator=NOT  Inputs=1
  Carrier Wave : simulink/Sources/Repeating Sequence  rep_seq_t=[0 1/(4*fc) 1/(2*fc) 3/(4*fc) 1/fc]  rep_seq_y=[0 1 0 -1 0]
  Carrier Wave1 : simulink/Sources/Repeating Sequence  rep_seq_t=[0 1/fc/4 3/fc/4 1/fc]  rep_seq_y=[0 -1 1 0]
  Constant : Constant  Value=m
  Data Type Conversion1 : DataTypeConversion  OutDataTypeStr=boolean
  Data Type Conversion2 : DataTypeConversion  OutDataTypeStr=boolean
  Data Type Conversion3 : DataTypeConversion  OutDataTypeStr=boolean
  Data Type Conversion4 : DataTypeConversion  OutDataTypeStr=double
  Mux : Mux  Inputs=6
  Product : Product
  Product1 : Product
  Product2 : Product
  Relational Operator : RelationalOperator
  Relational Operator1 : RelationalOperator
  Relational Operator2 : RelationalOperator
  Va : Sin  Frequency=2*pi*f  SampleTime=0
  Vb : Sin  Frequency=2*pi*f  Phase=-2*pi/3  SampleTime=0
  Vc : Sin  Frequency=2*pi*f  Phase=2*pi/3  SampleTime=0
  pwm : Outport  VectorParamsAs1DForOutWhenUnconnected=off
  wires:
  Constant/1 -> Product2/2, Product1/2, Product/2
  BL1/1 -> Mux/6
  Data Type Conversion2/1 -> BL5/1, Mux/3
  Vc/1 -> Product2/1
  Product/1 -> Relational Operator/1
  Data Type Conversion4/1 -> pwm/1
  Carrier Wave/1 -> Relational Operator1/2, Relational Operator/2, Relational Operator2/2
  BL5/1 -> Mux/4
  Relational Operator1/1 -> Data Type Conversion2/1
  Product1/1 -> Relational Operator1/1
  Relational Operator2/1 -> Data Type Conversion3/1
  Va/1 -> Product/1
  Data Type Conversion1/1 -> Mux/1, BL4/1
  Data Type Conversion3/1 -> Mux/5, BL1/1
  Vb/1 -> Product1/1
  BL4/1 -> Mux/2
  Product2/1 -> Relational Operator2/1
  Mux/1 -> Data Type Conversion4/1
  Relational Operator/1 -> Data Type Conversion1/1

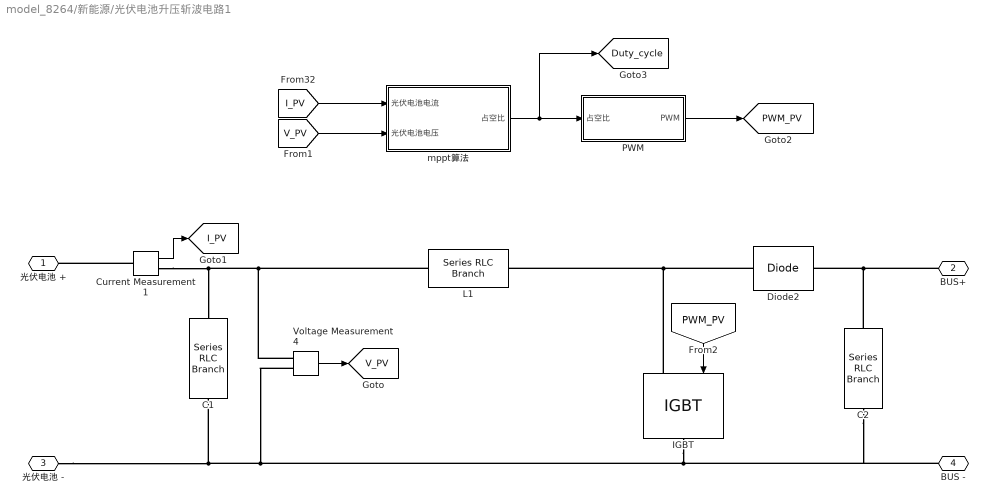
== system model_8264/新能源/光伏电池升压斩波电路1 ==
  C1 : spsSeriesRLCBranchLib/Series RLC Branch  LConnTagsString=__new0  RConnTagsString=__new0  BranchType=RC  Resistance=0.1  Inductance=1e-3  SetiL0=off  InitialCurrent=0  Capacitance=1e-3  Setx0=off  InitialVoltage=0  Measurements=None
  C2 : spsSeriesRLCBranchLib/Series RLC Branch  LConnTagsString=__new0  RConnTagsString=__new0  BranchType=C  Resistance=1  Inductance=1e-3  SetiL0=off  InitialCurrent=0  Capacitance=0.001  Setx0=off  InitialVoltage=0  Measurements=None
  Current Measurement1 : spsCurrentMeasurementLib/Current Measurement  PhasorSimulation=off  OutputType=Complex  PSBequivalent=0
  Diode2 : spsDiodeLib/Diode  Ron=0.001  Lon=0  Vf=0.8  IC=0  UseSnubber=0  Rs=inf  Cs=250e-9  Measurements=off
  IGBT : spsIGBTLib/IGBT  Ron=0.001  Lon=0  Vf=1  Tf=1e-6  Tt=2e-6  IC=0  Rs=1e5  Cs=inf  Measurements=off
  L1 : spsSeriesRLCBranchLib/Series RLC Branch  LConnTagsString=__new0  RConnTagsString=__new0  BranchType=L  Resistance=1  Inductance=1e-3  SetiL0=off  InitialCurrent=0  Capacitance=1e-6  Setx0=off  InitialVoltage=0  Measurements=None
  PWM : Subsystem
  Voltage Measurement4 : spsVoltageMeasurementLib/Voltage Measurement  PhasorSimulation=off  OutputType=Complex  PSBequivalent=0
  mppt算法 : Subsystem
  光伏电池 + : PMIOPort  Side=Left
  BUS+ : PMIOPort  Port=2  Side=Right
  光伏电池 - : PMIOPort  Port=3  Side=Left
  BUS - : PMIOPort  Port=4  Side=Right
  tag scope: Duty_cycle=global, I_PV=global, PWM_PV=global, V_PV=global
  wires:
  Voltage Measurement4/1 -> [V_PV]
  [I_PV] -> mppt算法/1(光伏电池电流)
  [V_PV] -> mppt算法/2(光伏电池电压)
  mppt算法/1(占空比) -> [Duty_cycle], PWM/1(占空比)
  PWM/1(PWM) -> [PWM_PV]
  [PWM_PV] -> IGBT/1
  Current Measurement1/1 -> [I_PV]
  connections:
  Voltage Measurement4/LConn1 -- L1/LConn1 -- C1/LConn1 -- Current Measurement1/RConn1
  光伏电池 -/RConn1 -- BUS -/RConn1 -- C2/RConn1 -- IGBT/RConn1 -- Voltage Measurement4/LConn2 -- C1/RConn1
  IGBT/LConn1 -- Diode2/LConn1 -- L1/RConn1
  C2/LConn1 -- BUS+/RConn1 -- Diode2/RConn1
  Current Measurement1/LConn1 -- 光伏电池 +/RConn1

== system model_8264/新能源/光照和温度控制1 ==
  Demux : Demux  Tag=STV Demux  Outputs=2
      settings: DisplayOption=none
  FromWs : FromWorkspace  Tag=STV FromWs  VariableName=tuvar
      SigBuilderData=|
      | common.afterFinalStr = 'Extrapolate'
      | common.sampleTime = 0
      | dataSet.timeRange = [0 5]
      | dataSet.name = 'Group 1'
      | sbobj.Groups.Name = 'Group 1'
      | sbobj.Groups.Signals(1).Name = 'Signal 1'
      | sbobj.Groups.Signals(1).XData = [0 0.5 0.5 5]
      | sbobj.Groups.Signals(1).YData = [100 100 1490 1490]
      | sbobj.Groups.Signals(2).Name = 'Signal 2'
      | sbobj.Groups.Signals(2).XData = [0 5]
      | sbobj.Groups.Signals(2).YData = [25 25]
      | sbobj.Groups.TimeRange = [0 5]
  Signal 1 : Outport  Tag=STV Outport
  Signal 2 : Outport  Tag=STV Outport  Port=2
  wires:
  Demux/1 -> Signal 1/1
  FromWs/1 -> Demux/1
  Demux/2 -> Signal 2/1

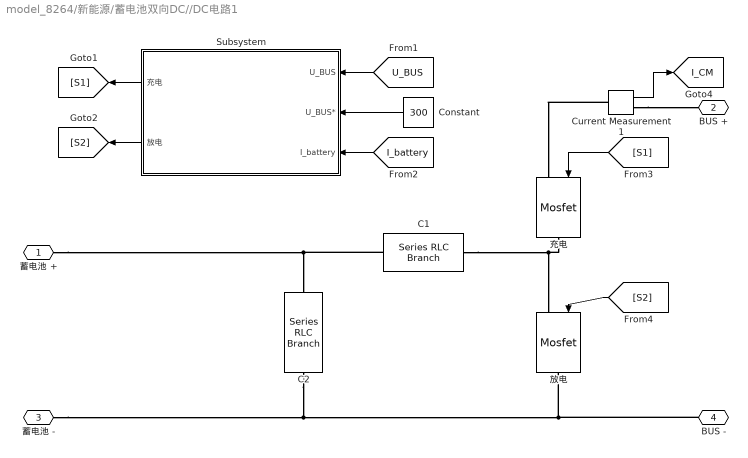
== system model_8264/新能源/蓄电池双向DC//DC电路1 ==
  C1 : spsSeriesRLCBranchLib/Series RLC Branch  LConnTagsString=__new0  RConnTagsString=__new0  BranchType=L  Resistance=0.1  Inductance=0.01  SetiL0=off  InitialCurrent=0  Capacitance=1e-3  Setx0=off  InitialVoltage=0  Measurements=None
  C2 : spsSeriesRLCBranchLib/Series RLC Branch  LConnTagsString=__new0  RConnTagsString=__new0  BranchType=RC  Resistance=0.1  Inductance=1e-3  SetiL0=off  InitialCurrent=0  Capacitance=1e-4  Setx0=off  InitialVoltage=0  Measurements=None
  Constant : Constant  Value=300
  Current Measurement1 : spsCurrentMeasurementLib/Current Measurement  PhasorSimulation=off  OutputType=Complex  PSBequivalent=0
  Subsystem : Subsystem
  充电 : spsMosfetLib/Mosfet  Ron=0.1  Lon=0  Rd=0.01  Vfd=0  IC=0  Rs=1e5  Cs=inf  Measurements=off
  放电 : spsMosfetLib/Mosfet  Ron=0.1  Lon=0  Rd=0.01  Vfd=0  IC=0  Rs=1e5  Cs=inf  Measurements=off
  蓄电池 + : PMIOPort  Side=Left
  BUS + : PMIOPort  Port=2  Side=Right
  蓄电池 - : PMIOPort  Port=3  Side=Left
  BUS - : PMIOPort  Port=4  Side=Right
  tag scope: I_CM=global
  wires:
  [U_BUS] -> Subsystem/1(U_BUS)
  [I_battery] -> Subsystem/3(I_battery)
  Constant/1 -> Subsystem/2(U_BUS*)
  Subsystem/1(充电) -> [S1]
  Subsystem/2(放电) -> [S2]
  [S1] -> 充电/1
  [S2] -> 放电/1
  Current Measurement1/1 -> [I_CM]
  connections:
  C2/RConn1 -- 蓄电池 -/RConn1 -- BUS -/RConn1 -- 放电/RConn1
  充电/RConn1 -- C1/LConn1 -- 放电/LConn1
  C1/RConn1 -- 蓄电池 +/RConn1 -- C2/LConn1
  Current Measurement1/LConn1 -- 充电/LConn1
  Current Measurement1/RConn1 -- BUS +/RConn1

== system model_8264/新负荷3/一天的时间曲线 ==
  Demux : Demux  Tag=STV Demux  Outputs=1
      settings: DisplayOption=none
  FromWs : FromWorkspace  Tag=STV FromWs  VariableName=tuvar
      SigBuilderData=|
      | common.afterFinalStr = 'Extrapolate'
      | common.sampleTime = 0
      | dataSet.timeRange = [0 24]
      | dataSet.name = 'Group 1'
      | sbobj.Groups.Name = 'Group 1'
      | sbobj.Groups.Signals.Name = 'Signal 1'
      | sbobj.Groups.Signals.XData = [0 0.01 0.02 0.03 0.04 0.05 0.06 0.07 0.08 0.09 0.1 0.11 0.12 0.13 0.14 0.15 0.16 0.17 0.18 0.19 0.2 0.21 0.22 0.23 0.24 0.25 0.26 0.27 0.28 0.29 0.3 0.31 0.32 0.33 0.34 0.35 0.36 0.37 0.38 0.39 0.4 0.41 0.42 0.43 0.44 0.45 0.46 0.47 0.48 0.49 0.5 0.51 0.52 0.53 0.54 0.55 0.56 0.57 0.58 0.59 0.6 0.61 0.62 0.63 0.64 0.65 0.66 0.67 0.68 0.69 0.7 0.71 0.72 0.73 0.74 0.75 0.76 0.77 0.78 0.79 0.8 0.81 0.82 0.83 0.84 0.85 0.86 0.87 0.88 0.89 0.9 0.91 0.92 0.93 0.94 0.95 0.96 0.97 0.98 0.99 1 1.01 1.02 1.03 1.04 1.05 1.06 1.07 1.08 1.09 1.1 1.11 1.12 1.13 1.14 1.15 1.16 1.17 1.18 1.19 1.2 1.21 1.22 1.23 1.24 1.25 1.26 1.27 1.28 1.29 1.3 1.31 1.32 1.33 1.34 1.35 1.36 1.37 1.38 1.39 1.4 1.41 1.42 1.43 1.44 1.45 1.46 1.47 1.48 1.49 1.5 1.51 1.52 1.53 1.54 1.55 1.56 1.57 1.58 1.59 1.6 1.61 1.62 1.63 1.64 1.65 1.66 1.67 1.68 1.69 1.7 1.71 1.72 1.73 1.74 1.75 1.76 1.77 1.78 1.79 1.8 1.81 1.82 1.83 1.84 1.85 1.86 1.87 1.88 1.89 1.9 1.91 1.92 1.93 1.94 1.95 1.96 1.97 1.98 1.99 2 2.01 2.02 2.03 2.04 2.05 2.06 2.07 2.08 2.09 2.1 2.11 2.12 2.13 2.14 2.15 2.16 2.17 2.18 2.19 2.2 2.21 2.22 2.23 2.24 2.25 2.26 2.27 2.28 2.29 2.3 2.31 2.32 2.33 2.34 2.35 2.36 2.37 2.38 2.39 2.4 24]
      | sbobj.Groups.Signals.YData = [0 0.01 0.02 0.03 0.04 0.05 0.06 0.07 0.08 0.09 0.1 0.11 0.12 0.13 0.14 0.15 0.16 0.17 0.18 0.19 0.2 0.21 0.22 0.23 0.24 0.25 0.26 0.27 0.28 0.29 0.3 0.31 0.32 0.33 0.34 0.35 0.36 0.37 0.38 0.39 0.4 0.41 0.42 0.43 0.44 0.45 0.46 0.47 0.48 0.49 0.5 0.51 0.52 0.53 0.54 0.55 0.56 0.57 0.58 0.59 0.6 0.61 0.62 0.63 0.64 0.65 0.66 0.67 0.68 0.69 0.7 0.71 0.72 0.73 0.74 0.75 0.76 0.77 0.78 0.79 0.8 0.81 0.82 0.83 0.84 0.85 0.86 0.87 0.88 0.89 0.9 0.91 0.92 0.93 0.94 0.95 0.96 0.97 0.98 0.99 1 1.01 1.02 1.03 1.04 1.05 1.06 1.07 1.08 1.09 1.1 1.11 1.12 1.13 1.14 1.15 1.16 1.17 1.18 1.19 1.2 1.21 1.22 1.23 1.24 1.25 1.26 1.27 1.28 1.29 1.3 1.31 1.32 1.33 1.34 1.35 1.36 1.37 1.38 1.39 1.4 1.41 1.42 1.43 1.44 1.45 1.46 1.47 1.48 1.49 1.5 1.51 1.52 1.53 1.54 1.55 1.56 1.57 1.58 1.59 1.6 1.61 1.62 1.63 1.64 1.65 1.66 1.67 1.68 1.69 1.7 1.71 1.72 1.73 1.74 1.75 1.76 1.77 1.78 1.79 1.8 1.81 1.82 1.83 1.84 1.85 1.86 1.87 1.88 1.89 1.9 1.91 1.92 1.93 1.94 1.95 1.96 1.97 1.98 1.99 2 2.01 2.02 2.03 2.04 2.05 2.06 2.07 2.08 2.09 2.1 2.11 2.12 2.13 2.14 2.15 2.16 2.17 2.18 2.19 2.2 2.21 2.22 2.23 2.24 2.25 2.26 2.27 2.28 2.29 2.3 2.31 2.32 2.33 2.34 2.35 2.36 2.37 2.38 2.39 2.4 2.4]
      | sbobj.Groups.TimeRange = [0 24]
  Signal 1 : Outport  Tag=STV Outport
  wires:
  FromWs/1 -> Demux/1
  Demux/1 -> Signal 1/1

== system model_8264/新负荷3/一天的时间曲线1 ==
  Demux : Demux  Tag=STV Demux  Outputs=1
      settings: DisplayOption=none
  FromWs : FromWorkspace  Tag=STV FromWs  VariableName=tuvar
      SigBuilderData=|
      | common.afterFinalStr = 'Extrapolate'
      | common.sampleTime = 0
      | dataSet.timeRange = [0 24]
      | dataSet.name = 'Group 1'
      | sbobj.Groups.Name = 'Group 1'
      | sbobj.Groups.Signals.Name = 'Signal 1'
      | sbobj.Groups.Signals.XData = [0 0.01 0.02 0.03 0.04 0.05 0.06 0.07 0.08 0.09 0.1 0.11 0.12 0.13 0.14 0.15 0.16 0.17 0.18 0.19 0.2 0.21 0.22 0.23 0.24 0.25 0.26 0.27 0.28 0.29 0.3 0.31 0.32 0.33 0.34 0.35 0.36 0.37 0.38 0.39 0.4 0.41 0.42 0.43 0.44 0.45 0.46 0.47 0.48 0.49 0.5 0.51 0.52 0.53 0.54 0.55 0.56 0.57 0.58 0.59 0.6 0.61 0.62 0.63 0.64 0.65 0.66 0.67 0.68 0.69 0.7 0.71 0.72 0.73 0.74 0.75 0.76 0.77 0.78 0.79 0.8 0.81 0.82 0.83 0.84 0.85 0.86 0.87 0.88 0.89 0.9 0.91 0.92 0.93 0.94 0.95 0.96 0.97 0.98 0.99 1 1.01 1.02 1.03 1.04 1.05 1.06 1.07 1.08 1.09 1.1 1.11 1.12 1.13 1.14 1.15 1.16 1.17 1.18 1.19 1.2 1.21 1.22 1.23 1.24 1.25 1.26 1.27 1.28 1.29 1.3 1.31 1.32 1.33 1.34 1.35 1.36 1.37 1.38 1.39 1.4 1.41 1.42 1.43 1.44 1.45 1.46 1.47 1.48 1.49 1.5 1.51 1.52 1.53 1.54 1.55 1.56 1.57 1.58 1.59 1.6 1.61 1.62 1.63 1.64 1.65 1.66 1.67 1.68 1.69 1.7 1.71 1.72 1.73 1.74 1.75 1.76 1.77 1.78 1.79 1.8 1.81 1.82 1.83 1.84 1.85 1.86 1.87 1.88 1.89 1.9 1.91 1.92 1.93 1.94 1.95 1.96 1.97 1.98 1.99 2 2.01 2.02 2.03 2.04 2.05 2.06 2.07 2.08 2.09 2.1 2.11 2.12 2.13 2.14 2.15 2.16 2.17 2.18 2.19 2.2 2.21 2.22 2.23 2.24 2.25 2.26 2.27 2.28 2.29 2.3 2.31 2.32 2.33 2.34 2.35 2.36 2.37 2.38 2.39 2.4 24]
      | sbobj.Groups.Signals.YData = [0 0.01 0.02 0.03 0.04 0.05 0.06 0.07 0.08 0.09 0.1 0.11 0.12 0.13 0.14 0.15 0.16 0.17 0.18 0.19 0.2 0.21 0.22 0.23 0.24 0.25 0.26 0.27 0.28 0.29 0.3 0.31 0.32 0.33 0.34 0.35 0.36 0.37 0.38 0.39 0.4 0.41 0.42 0.43 0.44 0.45 0.46 0.47 0.48 0.49 0.5 0.51 0.52 0.53 0.54 0.55 0.56 0.57 0.58 0.59 0.6 0.61 0.62 0.63 0.64 0.65 0.66 0.67 0.68 0.69 0.7 0.71 0.72 0.73 0.74 0.75 0.76 0.77 0.78 0.79 0.8 0.81 0.82 0.83 0.84 0.85 0.86 0.87 0.88 0.89 0.9 0.91 0.92 0.93 0.94 0.95 0.96 0.97 0.98 0.99 1 1.01 1.02 1.03 1.04 1.05 1.06 1.07 1.08 1.09 1.1 1.11 1.12 1.13 1.14 1.15 1.16 1.17 1.18 1.19 1.2 1.21 1.22 1.23 1.24 1.25 1.26 1.27 1.28 1.29 1.3 1.31 1.32 1.33 1.34 1.35 1.36 1.37 1.38 1.39 1.4 1.41 1.42 1.43 1.44 1.45 1.46 1.47 1.48 1.49 1.5 1.51 1.52 1.53 1.54 1.55 1.56 1.57 1.58 1.59 1.6 1.61 1.62 1.63 1.64 1.65 1.66 1.67 1.68 1.69 1.7 1.71 1.72 1.73 1.74 1.75 1.76 1.77 1.78 1.79 1.8 1.81 1.82 1.83 1.84 1.85 1.86 1.87 1.88 1.89 1.9 1.91 1.92 1.93 1.94 1.95 1.96 1.97 1.98 1.99 2 2.01 2.02 2.03 2.04 2.05 2.06 2.07 2.08 2.09 2.1 2.11 2.12 2.13 2.14 2.15 2.16 2.17 2.18 2.19 2.2 2.21 2.22 2.23 2.24 2.25 2.26 2.27 2.28 2.29 2.3 2.31 2.32 2.33 2.34 2.35 2.36 2.37 2.38 2.39 2.4 2.4]
      | sbobj.Groups.TimeRange = [0 24]
  Signal 1 : Outport  Tag=STV Outport
  wires:
  FromWs/1 -> Demux/1
  Demux/1 -> Signal 1/1

== system model_8264/新负荷3/一天的时间曲线2 ==
  Demux : Demux  Tag=STV Demux  Outputs=1
      settings: DisplayOption=none
  FromWs : FromWorkspace  Tag=STV FromWs  VariableName=tuvar
      SigBuilderData=|
      | common.afterFinalStr = 'Extrapolate'
      | common.sampleTime = 0
      | dataSet.timeRange = [0 24]
      | dataSet.name = 'Group 1'
      | sbobj.Groups.Name = 'Group 1'
      | sbobj.Groups.Signals.Name = 'Signal 1'
      | sbobj.Groups.Signals.XData = [0 0.01 0.02 0.03 0.04 0.05 0.06 0.07 0.08 0.09 0.1 0.11 0.12 0.13 0.14 0.15 0.16 0.17 0.18 0.19 0.2 0.21 0.22 0.23 0.24 0.25 0.26 0.27 0.28 0.29 0.3 0.31 0.32 0.33 0.34 0.35 0.36 0.37 0.38 0.39 0.4 0.41 0.42 0.43 0.44 0.45 0.46 0.47 0.48 0.49 0.5 0.51 0.52 0.53 0.54 0.55 0.56 0.57 0.58 0.59 0.6 0.61 0.62 0.63 0.64 0.65 0.66 0.67 0.68 0.69 0.7 0.71 0.72 0.73 0.74 0.75 0.76 0.77 0.78 0.79 0.8 0.81 0.82 0.83 0.84 0.85 0.86 0.87 0.88 0.89 0.9 0.91 0.92 0.93 0.94 0.95 0.96 0.97 0.98 0.99 1 1.01 1.02 1.03 1.04 1.05 1.06 1.07 1.08 1.09 1.1 1.11 1.12 1.13 1.14 1.15 1.16 1.17 1.18 1.19 1.2 1.21 1.22 1.23 1.24 1.25 1.26 1.27 1.28 1.29 1.3 1.31 1.32 1.33 1.34 1.35 1.36 1.37 1.38 1.39 1.4 1.41 1.42 1.43 1.44 1.45 1.46 1.47 1.48 1.49 1.5 1.51 1.52 1.53 1.54 1.55 1.56 1.57 1.58 1.59 1.6 1.61 1.62 1.63 1.64 1.65 1.66 1.67 1.68 1.69 1.7 1.71 1.72 1.73 1.74 1.75 1.76 1.77 1.78 1.79 1.8 1.81 1.82 1.83 1.84 1.85 1.86 1.87 1.88 1.89 1.9 1.91 1.92 1.93 1.94 1.95 1.96 1.97 1.98 1.99 2 2.01 2.02 2.03 2.04 2.05 2.06 2.07 2.08 2.09 2.1 2.11 2.12 2.13 2.14 2.15 2.16 2.17 2.18 2.19 2.2 2.21 2.22 2.23 2.24 2.25 2.26 2.27 2.28 2.29 2.3 2.31 2.32 2.33 2.34 2.35 2.36 2.37 2.38 2.39 2.4 24]
      | sbobj.Groups.Signals.YData = [0 0.01 0.02 0.03 0.04 0.05 0.06 0.07 0.08 0.09 0.1 0.11 0.12 0.13 0.14 0.15 0.16 0.17 0.18 0.19 0.2 0.21 0.22 0.23 0.24 0.25 0.26 0.27 0.28 0.29 0.3 0.31 0.32 0.33 0.34 0.35 0.36 0.37 0.38 0.39 0.4 0.41 0.42 0.43 0.44 0.45 0.46 0.47 0.48 0.49 0.5 0.51 0.52 0.53 0.54 0.55 0.56 0.57 0.58 0.59 0.6 0.61 0.62 0.63 0.64 0.65 0.66 0.67 0.68 0.69 0.7 0.71 0.72 0.73 0.74 0.75 0.76 0.77 0.78 0.79 0.8 0.81 0.82 0.83 0.84 0.85 0.86 0.87 0.88 0.89 0.9 0.91 0.92 0.93 0.94 0.95 0.96 0.97 0.98 0.99 1 1.01 1.02 1.03 1.04 1.05 1.06 1.07 1.08 1.09 1.1 1.11 1.12 1.13 1.14 1.15 1.16 1.17 1.18 1.19 1.2 1.21 1.22 1.23 1.24 1.25 1.26 1.27 1.28 1.29 1.3 1.31 1.32 1.33 1.34 1.35 1.36 1.37 1.38 1.39 1.4 1.41 1.42 1.43 1.44 1.45 1.46 1.47 1.48 1.49 1.5 1.51 1.52 1.53 1.54 1.55 1.56 1.57 1.58 1.59 1.6 1.61 1.62 1.63 1.64 1.65 1.66 1.67 1.68 1.69 1.7 1.71 1.72 1.73 1.74 1.75 1.76 1.77 1.78 1.79 1.8 1.81 1.82 1.83 1.84 1.85 1.86 1.87 1.88 1.89 1.9 1.91 1.92 1.93 1.94 1.95 1.96 1.97 1.98 1.99 2 2.01 2.02 2.03 2.04 2.05 2.06 2.07 2.08 2.09 2.1 2.11 2.12 2.13 2.14 2.15 2.16 2.17 2.18 2.19 2.2 2.21 2.22 2.23 2.24 2.25 2.26 2.27 2.28 2.29 2.3 2.31 2.32 2.33 2.34 2.35 2.36 2.37 2.38 2.39 2.4 2.4]
      | sbobj.Groups.TimeRange = [0 24]
  Signal 1 : Outport  Tag=STV Outport
  wires:
  FromWs/1 -> Demux/1
  Demux/1 -> Signal 1/1

== system model_8264/新负荷3/洗衣机(1000W) ==
  note: 电源
  note: 开关信号
      | 0:负载断开
      | 1:负载接上
  y : Inport
  Current Measurement1 : spsCurrentMeasurementLib/Current Measurement  PhasorSimulation=off  OutputType=Complex  PSBequivalent=0
  Ground1 : spsGroundLib/Ground  LConnTagsString=a
  Ideal Switch : spsIdealSwitchLib/Ideal Switch  Ron=0.001  Lon=0  IC=0  Rs=1e5  Cs=inf  Measurements=off
  Mean : spsMeanLib/Mean  Freq=50  Vinit=0  Ts=0
  Product : Product
  Series RLC Load : spsSeriesRLCLoadLib/Series RLC Load  LConnTagsString=a  RConnTagsString=__new0  NominalVoltage=220  NominalFrequency=50  ActivePower=5000  InductivePower=100  CapacitivePower=100  Setx0=off  InitialVoltage=0  SetiL0=off  InitialCurrent=0  Measurements=None  LoadType=constant Z
  Voltage Measurement2 : spsVoltageMeasurementLib/Voltage Measurement  PhasorSimulation=off  OutputType=Complex  PSBequivalent=0
  Connection Port : PMIOPort  Side=Left
  P : Outport
  wires:
  y/1 -> Ideal Switch/1
  Voltage Measurement2/1 -> Product/1
  Current Measurement1/1 -> Product/2
  Product/1 -> Mean/1
  Mean/1 -> P/1
  connections:
  Series RLC Load/LConn1 -- Ideal Switch/RConn1 -- Voltage Measurement2/LConn1
  Ideal Switch/LConn1 -- Connection Port/RConn1
  Current Measurement1/LConn1 -- Series RLC Load/RConn1
  Voltage Measurement2/LConn2 -- Current Measurement1/RConn1 -- Ground1/LConn1

== system model_8264/新负荷3/洗衣机(1000W)1 ==
  note: 电源
  note: 开关信号
      | 0:负载断开
      | 1:负载接上
  y : Inport
  Current Measurement1 : spsCurrentMeasurementLib/Current Measurement  PhasorSimulation=off  OutputType=Complex  PSBequivalent=0
  Ground1 : spsGroundLib/Ground  LConnTagsString=a
  Ideal Switch : spsIdealSwitchLib/Ideal Switch  Ron=0.001  Lon=0  IC=0  Rs=1e5  Cs=inf  Measurements=off
  Mean : spsMeanLib/Mean  Freq=50  Vinit=0  Ts=0
  Product : Product
  Series RLC Load : spsSeriesRLCLoadLib/Series RLC Load  LConnTagsString=a  RConnTagsString=__new0  NominalVoltage=220  NominalFrequency=50  ActivePower=5000  InductivePower=100  CapacitivePower=100  Setx0=off  InitialVoltage=0  SetiL0=off  InitialCurrent=0  Measurements=None  LoadType=constant Z
  Voltage Measurement2 : spsVoltageMeasurementLib/Voltage Measurement  PhasorSimulation=off  OutputType=Complex  PSBequivalent=0
  Connection Port : PMIOPort  Side=Left
  P : Outport
  wires:
  y/1 -> Ideal Switch/1
  Voltage Measurement2/1 -> Product/1
  Current Measurement1/1 -> Product/2
  Product/1 -> Mean/1
  Mean/1 -> P/1
  connections:
  Series RLC Load/LConn1 -- Ideal Switch/RConn1 -- Voltage Measurement2/LConn1
  Ideal Switch/LConn1 -- Connection Port/RConn1
  Current Measurement1/LConn1 -- Series RLC Load/RConn1
  Voltage Measurement2/LConn2 -- Current Measurement1/RConn1 -- Ground1/LConn1

== system model_8264/新负荷3/洗衣机(1000W)2 ==
  note: 电源
  note: 开关信号
      | 0:负载断开
      | 1:负载接上
  y : Inport
  Current Measurement1 : spsCurrentMeasurementLib/Current Measurement  PhasorSimulation=off  OutputType=Complex  PSBequivalent=0
  Ground1 : spsGroundLib/Ground  LConnTagsString=a
  Ideal Switch : spsIdealSwitchLib/Ideal Switch  Ron=0.001  Lon=0  IC=0  Rs=1e5  Cs=inf  Measurements=off
  Mean : spsMeanLib/Mean  Freq=50  Vinit=0  Ts=0
  Product : Product
  Series RLC Load : spsSeriesRLCLoadLib/Series RLC Load  LConnTagsString=a  RConnTagsString=__new0  NominalVoltage=220  NominalFrequency=50  ActivePower=5000  InductivePower=100  CapacitivePower=100  Setx0=off  InitialVoltage=0  SetiL0=off  InitialCurrent=0  Measurements=None  LoadType=constant Z
  Voltage Measurement2 : spsVoltageMeasurementLib/Voltage Measurement  PhasorSimulation=off  OutputType=Complex  PSBequivalent=0
  Connection Port : PMIOPort  Side=Left
  P : Outport
  wires:
  y/1 -> Ideal Switch/1
  Voltage Measurement2/1 -> Product/1
  Current Measurement1/1 -> Product/2
  Product/1 -> Mean/1
  Mean/1 -> P/1
  connections:
  Series RLC Load/LConn1 -- Ideal Switch/RConn1 -- Voltage Measurement2/LConn1
  Ideal Switch/LConn1 -- Connection Port/RConn1
  Current Measurement1/LConn1 -- Series RLC Load/RConn1
  Voltage Measurement2/LConn2 -- Current Measurement1/RConn1 -- Ground1/LConn1

== system model_8264/新负荷3/电灯(60W) ==
  note: 电源
  note: 开关信号
      | 0:负载断开
      | 1:负载接上
  y : Inport
  Current Measurement1 : spsCurrentMeasurementLib/Current Measurement  PhasorSimulation=off  OutputType=Complex  PSBequivalent=0
  Ground1 : spsGroundLib/Ground  LConnTagsString=a
  Ideal Switch : spsIdealSwitchLib/Ideal Switch  Ron=0.001  Lon=0  IC=0  Rs=1e5  Cs=inf  Measurements=off
  Mean : spsMeanLib/Mean  Freq=50  Vinit=0  Ts=0
  Product : Product
  Series RLC Load : spsSeriesRLCLoadLib/Series RLC Load  LConnTagsString=a  RConnTagsString=__new0  NominalVoltage=220  NominalFrequency=50  ActivePower=600  InductivePower=100  CapacitivePower=100  Setx0=off  InitialVoltage=0  SetiL0=off  InitialCurrent=0  Measurements=None  LoadType=constant Z
  Voltage Measurement2 : spsVoltageMeasurementLib/Voltage Measurement  PhasorSimulation=off  OutputType=Complex  PSBequivalent=0
  Connection Port : PMIOPort  Side=Left
  P : Outport
  wires:
  y/1 -> Ideal Switch/1
  Voltage Measurement2/1 -> Product/1
  Current Measurement1/1 -> Product/2
  Product/1 -> Mean/1
  Mean/1 -> P/1
  connections:
  Ideal Switch/RConn1 -- Voltage Measurement2/LConn1 -- Series RLC Load/LConn1
  Ideal Switch/LConn1 -- Connection Port/RConn1
  Current Measurement1/LConn1 -- Series RLC Load/RConn1
  Current Measurement1/RConn1 -- Ground1/LConn1 -- Voltage Measurement2/LConn2

== system model_8264/新负荷3/电灯(60W)1 ==
  note: 电源
  note: 开关信号
      | 0:负载断开
      | 1:负载接上
  y : Inport
  Current Measurement1 : spsCurrentMeasurementLib/Current Measurement  PhasorSimulation=off  OutputType=Complex  PSBequivalent=0
  Ground1 : spsGroundLib/Ground  LConnTagsString=a
  Ideal Switch : spsIdealSwitchLib/Ideal Switch  Ron=0.001  Lon=0  IC=0  Rs=1e5  Cs=inf  Measurements=off
  Mean : spsMeanLib/Mean  Freq=50  Vinit=0  Ts=0
  Product : Product
  Series RLC Load : spsSeriesRLCLoadLib/Series RLC Load  LConnTagsString=a  RConnTagsString=__new0  NominalVoltage=220  NominalFrequency=50  ActivePower=600  InductivePower=100  CapacitivePower=100  Setx0=off  InitialVoltage=0  SetiL0=off  InitialCurrent=0  Measurements=None  LoadType=constant Z
  Voltage Measurement2 : spsVoltageMeasurementLib/Voltage Measurement  PhasorSimulation=off  OutputType=Complex  PSBequivalent=0
  Connection Port : PMIOPort  Side=Left
  P : Outport
  wires:
  y/1 -> Ideal Switch/1
  Voltage Measurement2/1 -> Product/1
  Current Measurement1/1 -> Product/2
  Product/1 -> Mean/1
  Mean/1 -> P/1
  connections:
  Ideal Switch/RConn1 -- Voltage Measurement2/LConn1 -- Series RLC Load/LConn1
  Ideal Switch/LConn1 -- Connection Port/RConn1
  Current Measurement1/LConn1 -- Series RLC Load/RConn1
  Current Measurement1/RConn1 -- Ground1/LConn1 -- Voltage Measurement2/LConn2

== system model_8264/新负荷3/电灯(60W)2 ==
  note: 电源
  note: 开关信号
      | 0:负载断开
      | 1:负载接上
  y : Inport
  Current Measurement1 : spsCurrentMeasurementLib/Current Measurement  PhasorSimulation=off  OutputType=Complex  PSBequivalent=0
  Ground1 : spsGroundLib/Ground  LConnTagsString=a
  Ideal Switch : spsIdealSwitchLib/Ideal Switch  Ron=0.001  Lon=0  IC=0  Rs=1e5  Cs=inf  Measurements=off
  Mean : spsMeanLib/Mean  Freq=50  Vinit=0  Ts=0
  Product : Product
  Series RLC Load : spsSeriesRLCLoadLib/Series RLC Load  LConnTagsString=a  RConnTagsString=__new0  NominalVoltage=220  NominalFrequency=50  ActivePower=600  InductivePower=100  CapacitivePower=100  Setx0=off  InitialVoltage=0  SetiL0=off  InitialCurrent=0  Measurements=None  LoadType=constant Z
  Voltage Measurement2 : spsVoltageMeasurementLib/Voltage Measurement  PhasorSimulation=off  OutputType=Complex  PSBequivalent=0
  Connection Port : PMIOPort  Side=Left
  P : Outport
  wires:
  y/1 -> Ideal Switch/1
  Voltage Measurement2/1 -> Product/1
  Current Measurement1/1 -> Product/2
  Product/1 -> Mean/1
  Mean/1 -> P/1
  connections:
  Ideal Switch/RConn1 -- Voltage Measurement2/LConn1 -- Series RLC Load/LConn1
  Ideal Switch/LConn1 -- Connection Port/RConn1
  Current Measurement1/LConn1 -- Series RLC Load/RConn1
  Current Measurement1/RConn1 -- Ground1/LConn1 -- Voltage Measurement2/LConn2

== system model_8264/新负荷3/电饭锅(800W) ==
  note: 电源
  note: 开关信号
      | 0:负载断开
      | 1:负载接上
  y : Inport
  Current Measurement1 : spsCurrentMeasurementLib/Current Measurement  PhasorSimulation=off  OutputType=Complex  PSBequivalent=0
  Ground1 : spsGroundLib/Ground  LConnTagsString=a
  Ideal Switch : spsIdealSwitchLib/Ideal Switch  Ron=0.001  Lon=0  IC=0  Rs=1e5  Cs=inf  Measurements=off
  Mean : spsMeanLib/Mean  Freq=50  Vinit=0  Ts=0
  Product : Product
  Series RLC Load : spsSeriesRLCLoadLib/Series RLC Load  LConnTagsString=a  RConnTagsString=__new0  NominalVoltage=400  NominalFrequency=50  ActivePower=8000  InductivePower=100  CapacitivePower=100  Setx0=off  InitialVoltage=0  SetiL0=off  InitialCurrent=0  Measurements=None  LoadType=constant Z
  Voltage Measurement2 : spsVoltageMeasurementLib/Voltage Measurement  PhasorSimulation=off  OutputType=Complex  PSBequivalent=0
  Connection Port : PMIOPort  Side=Left
  P : Outport
  wires:
  y/1 -> Ideal Switch/1
  Voltage Measurement2/1 -> Product/1
  Current Measurement1/1 -> Product/2
  Product/1 -> Mean/1
  Mean/1 -> P/1
  connections:
  Series RLC Load/LConn1 -- Ideal Switch/RConn1 -- Voltage Measurement2/LConn1
  Ideal Switch/LConn1 -- Connection Port/RConn1
  Current Measurement1/LConn1 -- Series RLC Load/RConn1
  Voltage Measurement2/LConn2 -- Current Measurement1/RConn1 -- Ground1/LConn1

== system model_8264/新负荷3/电饭锅(800W)1 ==
  note: 电源
  note: 开关信号
      | 0:负载断开
      | 1:负载接上
  y : Inport
  Current Measurement1 : spsCurrentMeasurementLib/Current Measurement  PhasorSimulation=off  OutputType=Complex  PSBequivalent=0
  Ground1 : spsGroundLib/Ground  LConnTagsString=a
  Ideal Switch : spsIdealSwitchLib/Ideal Switch  Ron=0.001  Lon=0  IC=0  Rs=1e5  Cs=inf  Measurements=off
  Mean : spsMeanLib/Mean  Freq=50  Vinit=0  Ts=0
  Product : Product
  Series RLC Load : spsSeriesRLCLoadLib/Series RLC Load  LConnTagsString=a  RConnTagsString=__new0  NominalVoltage=400  NominalFrequency=50  ActivePower=8000  InductivePower=100  CapacitivePower=100  Setx0=off  InitialVoltage=0  SetiL0=off  InitialCurrent=0  Measurements=None  LoadType=constant Z
  Voltage Measurement2 : spsVoltageMeasurementLib/Voltage Measurement  PhasorSimulation=off  OutputType=Complex  PSBequivalent=0
  Connection Port : PMIOPort  Side=Left
  P : Outport
  wires:
  y/1 -> Ideal Switch/1
  Voltage Measurement2/1 -> Product/1
  Current Measurement1/1 -> Product/2
  Product/1 -> Mean/1
  Mean/1 -> P/1
  connections:
  Series RLC Load/LConn1 -- Ideal Switch/RConn1 -- Voltage Measurement2/LConn1
  Ideal Switch/LConn1 -- Connection Port/RConn1
  Current Measurement1/LConn1 -- Series RLC Load/RConn1
  Voltage Measurement2/LConn2 -- Current Measurement1/RConn1 -- Ground1/LConn1

== system model_8264/新负荷3/电饭锅(800W)2 ==
  note: 电源
  note: 开关信号
      | 0:负载断开
      | 1:负载接上
  y : Inport
  Current Measurement1 : spsCurrentMeasurementLib/Current Measurement  PhasorSimulation=off  OutputType=Complex  PSBequivalent=0
  Ground1 : spsGroundLib/Ground  LConnTagsString=a
  Ideal Switch : spsIdealSwitchLib/Ideal Switch  Ron=0.001  Lon=0  IC=0  Rs=1e5  Cs=inf  Measurements=off
  Mean : spsMeanLib/Mean  Freq=50  Vinit=0  Ts=0
  Product : Product
  Series RLC Load : spsSeriesRLCLoadLib/Series RLC Load  LConnTagsString=a  RConnTagsString=__new0  NominalVoltage=400  NominalFrequency=50  ActivePower=8000  InductivePower=100  CapacitivePower=100  Setx0=off  InitialVoltage=0  SetiL0=off  InitialCurrent=0  Measurements=None  LoadType=constant Z
  Voltage Measurement2 : spsVoltageMeasurementLib/Voltage Measurement  PhasorSimulation=off  OutputType=Complex  PSBequivalent=0
  Connection Port : PMIOPort  Side=Left
  P : Outport
  wires:
  y/1 -> Ideal Switch/1
  Voltage Measurement2/1 -> Product/1
  Current Measurement1/1 -> Product/2
  Product/1 -> Mean/1
  Mean/1 -> P/1
  connections:
  Series RLC Load/LConn1 -- Ideal Switch/RConn1 -- Voltage Measurement2/LConn1
  Ideal Switch/LConn1 -- Connection Port/RConn1
  Current Measurement1/LConn1 -- Series RLC Load/RConn1
  Voltage Measurement2/LConn2 -- Current Measurement1/RConn1 -- Ground1/LConn1

== system model_8264/新负荷3/空调(1000W) ==
  note: 电源
  note: 开关信号
      | 0:负载断开
      | 1:负载接上
  y : Inport
  Current Measurement1 : spsCurrentMeasurementLib/Current Measurement  PhasorSimulation=off  OutputType=Complex  PSBequivalent=0
  Ground1 : spsGroundLib/Ground  LConnTagsString=a
  Ideal Switch : spsIdealSwitchLib/Ideal Switch  Ron=0.001  Lon=0  IC=0  Rs=1e5  Cs=inf  Measurements=off
  Mean : spsMeanLib/Mean  Freq=50  Vinit=0  Ts=0
  Product : Product
  Series RLC Load : spsSeriesRLCLoadLib/Series RLC Load  LConnTagsString=a  RConnTagsString=__new0  NominalVoltage=220  NominalFrequency=50  ActivePower=10000  InductivePower=100  CapacitivePower=100  Setx0=off  InitialVoltage=0  SetiL0=off  InitialCurrent=0  Measurements=None  LoadType=constant Z
  Voltage Measurement2 : spsVoltageMeasurementLib/Voltage Measurement  PhasorSimulation=off  OutputType=Complex  PSBequivalent=0
  Connection Port : PMIOPort  Side=Left
  P : Outport
  wires:
  y/1 -> Ideal Switch/1
  Voltage Measurement2/1 -> Product/1
  Current Measurement1/1 -> Product/2
  Product/1 -> Mean/1
  Mean/1 -> P/1
  connections:
  Series RLC Load/LConn1 -- Ideal Switch/RConn1 -- Voltage Measurement2/LConn1
  Ideal Switch/LConn1 -- Connection Port/RConn1
  Current Measurement1/LConn1 -- Series RLC Load/RConn1
  Voltage Measurement2/LConn2 -- Current Measurement1/RConn1 -- Ground1/LConn1

== system model_8264/新负荷3/空调(1000W)1 ==
  note: 电源
  note: 开关信号
      | 0:负载断开
      | 1:负载接上
  y : Inport
  Current Measurement1 : spsCurrentMeasurementLib/Current Measurement  PhasorSimulation=off  OutputType=Complex  PSBequivalent=0
  Ground1 : spsGroundLib/Ground  LConnTagsString=a
  Ideal Switch : spsIdealSwitchLib/Ideal Switch  Ron=0.001  Lon=0  IC=0  Rs=1e5  Cs=inf  Measurements=off
  Mean : spsMeanLib/Mean  Freq=50  Vinit=0  Ts=0
  Product : Product
  Series RLC Load : spsSeriesRLCLoadLib/Series RLC Load  LConnTagsString=a  RConnTagsString=__new0  NominalVoltage=220  NominalFrequency=50  ActivePower=10000  InductivePower=100  CapacitivePower=100  Setx0=off  InitialVoltage=0  SetiL0=off  InitialCurrent=0  Measurements=None  LoadType=constant Z
  Voltage Measurement2 : spsVoltageMeasurementLib/Voltage Measurement  PhasorSimulation=off  OutputType=Complex  PSBequivalent=0
  Connection Port : PMIOPort  Side=Left
  P : Outport
  wires:
  y/1 -> Ideal Switch/1
  Voltage Measurement2/1 -> Product/1
  Current Measurement1/1 -> Product/2
  Product/1 -> Mean/1
  Mean/1 -> P/1
  connections:
  Series RLC Load/LConn1 -- Ideal Switch/RConn1 -- Voltage Measurement2/LConn1
  Ideal Switch/LConn1 -- Connection Port/RConn1
  Current Measurement1/LConn1 -- Series RLC Load/RConn1
  Voltage Measurement2/LConn2 -- Current Measurement1/RConn1 -- Ground1/LConn1

== system model_8264/新负荷3/空调(1000W)2 ==
  note: 电源
  note: 开关信号
      | 0:负载断开
      | 1:负载接上
  y : Inport
  Current Measurement1 : spsCurrentMeasurementLib/Current Measurement  PhasorSimulation=off  OutputType=Complex  PSBequivalent=0
  Ground1 : spsGroundLib/Ground  LConnTagsString=a
  Ideal Switch : spsIdealSwitchLib/Ideal Switch  Ron=0.001  Lon=0  IC=0  Rs=1e5  Cs=inf  Measurements=off
  Mean : spsMeanLib/Mean  Freq=50  Vinit=0  Ts=0
  Product : Product
  Series RLC Load : spsSeriesRLCLoadLib/Series RLC Load  LConnTagsString=a  RConnTagsString=__new0  NominalVoltage=220  NominalFrequency=50  ActivePower=10000  InductivePower=100  CapacitivePower=100  Setx0=off  InitialVoltage=0  SetiL0=off  InitialCurrent=0  Measurements=None  LoadType=constant Z
  Voltage Measurement2 : spsVoltageMeasurementLib/Voltage Measurement  PhasorSimulation=off  OutputType=Complex  PSBequivalent=0
  Connection Port : PMIOPort  Side=Left
  P : Outport
  wires:
  y/1 -> Ideal Switch/1
  Voltage Measurement2/1 -> Product/1
  Current Measurement1/1 -> Product/2
  Product/1 -> Mean/1
  Mean/1 -> P/1
  connections:
  Series RLC Load/LConn1 -- Ideal Switch/RConn1 -- Voltage Measurement2/LConn1
  Ideal Switch/LConn1 -- Connection Port/RConn1
  Current Measurement1/LConn1 -- Series RLC Load/RConn1
  Voltage Measurement2/LConn2 -- Current Measurement1/RConn1 -- Ground1/LConn1

== system model_8264/新能源/光伏电池升压斩波电路1/PWM ==
  占空比 : Inport
  Constant : Constant
  Constant1 : Constant  Value=0
  Repeating Sequence : simulink/Sources/Repeating Sequence  rep_seq_t=[0 1e-4]  rep_seq_y=[0 2]
  Saturation : Saturate  UpperLimit=1  LowerLimit=0
  Scope : Scope  NumInputPorts=2
  Sum : Sum  Inputs=|+-
  Switch : Switch  Criteria=u2 > Threshold  SaturateOnIntegerOverflow=off  InputSameDT=off
  Zero-Order Hold : ZeroOrderHold  SampleTime=0.05
  PWM : Outport
  wires:
  占空比/1 -> Zero-Order Hold/1
  Zero-Order Hold/1 -> Saturation/1
  Switch/1 -> Scope/1, PWM/1
  Constant/1 -> Switch/1
  Constant1/1 -> Switch/3
  Saturation/1 -> Sum/1
  Sum/1 -> Switch/2
  Repeating Sequence/1 -> Scope/2, Sum/2
